simulink model "pendulo_invertido_bloque"  (R2025a)
settings: Solver=VariableStepAuto  StartTime=0.0  StopTime=10.0  RelTol=1e-3
PreLoadFcn:
  | % Parámetros físicos
  | Ip   = 0.0079;     % kg*m^2
  | Mc   = 0.7031;     % kg
  | lp   = 0.3302;     % m
  | lp2  = lp^2;       % m^2
  | lp3  = lp^3;       % m^3
  | Mp   = 0.23;       % kg
  | Mp2  = Mp^2;       % kg^2
  | Fc   = 0;          % N
  | Beq  = 4.3;        % Ns/m
  | g    = 9.81;       % m/s^2
  | Bp   = 0.0024;     % Nms/rad
  | 
  | % Condiciones iniciales de los estados
  | x       = 0;          % m
  | xdot      = 0;          % m/s
  | alpha   = 1*pi/180;   % rad
  | adot     = 0;          % rad/s
settings Model: Creator=Chris  LastModifiedBy=Chris

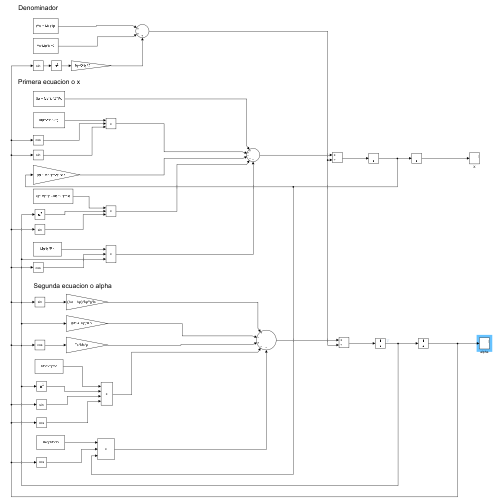
[thumbnail: Simulink's stored preview of the top-level diagram]
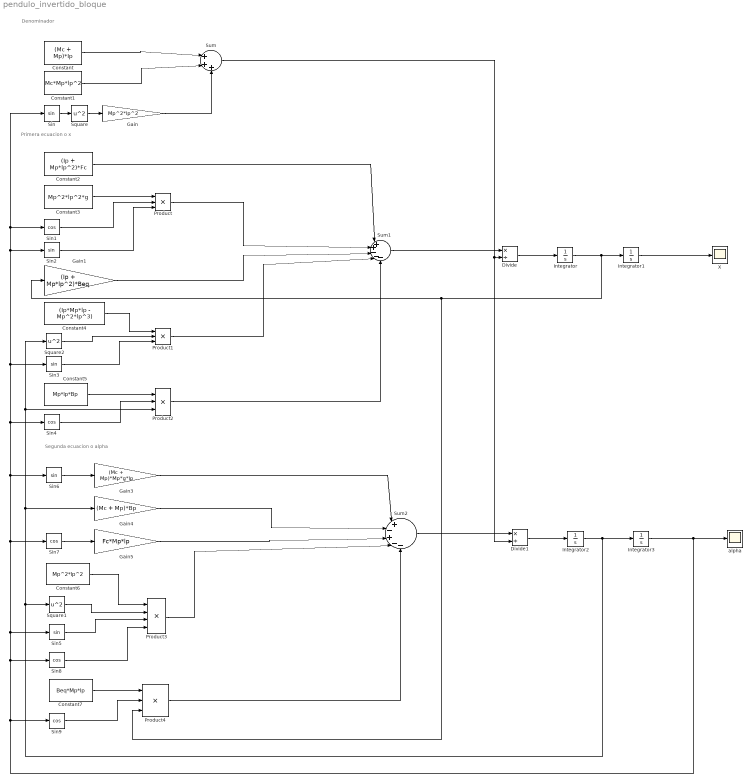
== system pendulo_invertido_bloque ==
  note: Segunda ecuacion o alpha
  note: Denominador
  note: Primera ecuacion o x
  Constant : Constant  Value=(Mc + Mp)*Ip
  Constant1 : Constant  Value=Mc*Mp*lp^2
  Constant2 : Constant  Value=(Ip + Mp*lp^2)*Fc
  Constant3 : Constant  Value=Mp^2*lp^2*g
  Constant4 : Constant  Value=(Ip*Mp*lp - Mp^2*lp^3)
  Constant5 : Constant  Value=Mp*lp*Bp
  Constant6 : Constant  Value=Mp^2*lp^2
  Constant7 : Constant  Value=Beq*Mp*lp
  Divide : Product  Inputs=*/
  Divide1 : Product  Inputs=*/
  Gain : Gain  Gain=Mp^2*lp^2
  Gain1 : Gain  Gain=(Ip + Mp*lp^2)*Beq
  Gain3 : Gain  Gain=(Mc + Mp)*Mp*g*lp
  Gain4 : Gain  Gain=(Mc + Mp)*Bp
  Gain5 : Gain  Gain=Fc*Mp*lp
  Integrator : Integrator
  Integrator1 : Integrator
  Integrator2 : Integrator
  Integrator3 : Integrator  InitialCondition=(1*pi)/180
  Product{,1..2,4} (4 alike) : Product  Inputs=3
  Product3 : Product  Inputs=4
  Sin{,2..3,5..6} (5 alike) : Trigonometry
  Sin{1,4,7..9} (5 alike) : Trigonometry  Operator=cos
  Square : Math  Operator=square
  Square1 : Math  Operator=square
  Square2 : Math  Operator=square
  Sum : Sum  Inputs=|+++
  Sum1 : Sum  Inputs=|++---
  Sum2 : Sum  Inputs=|+-+--
  X : Scope
      settings: ActiveDisplayYMinimum=-0.0043680008391681624  ActiveDisplayYMaximum=0.21434857965637735
  alpha : Scope
      settings: MaximizeAxes=On  ActiveDisplayYMinimum=-18.099425830783975  ActiveDisplayYMaximum=112.07325868766492
  wires:
  Constant/1 -> Sum/1
  Constant1/1 -> Sum/2
  Sin/1 -> Square/1
  Square/1 -> Gain/1
  Gain/1 -> Sum/3
  Constant2/1 -> Sum1/1
  Sin1/1 -> Product/2
  Constant3/1 -> Product/1
  Sin2/1 -> Product/3
  Product/1 -> Sum1/2
  Gain1/1 -> Sum1/3
  Constant4/1 -> Product1/1
  Square2/1 -> Product1/2
  Sin3/1 -> Product1/3
  Product1/1 -> Sum1/4
  Constant5/1 -> Product2/1
  Sin4/1 -> Product2/2
  Product2/1 -> Sum1/5
  Sin6/1 -> Gain3/1
  Sin7/1 -> Gain5/1
  Constant6/1 -> Product3/1
  Square1/1 -> Product3/2
  Sin5/1 -> Product3/3
  Sin8/1 -> Product3/4
  Constant7/1 -> Product4/1
  Sin9/1 -> Product4/2
  Gain3/1 -> Sum2/1
  Gain4/1 -> Sum2/2
  Gain5/1 -> Sum2/3
  Product3/1 -> Sum2/4
  Product4/1 -> Sum2/5
  Sum/1 -> Divide1/2, Divide/2
  Sum1/1 -> Divide/1
  Sum2/1 -> Divide1/1
  Divide/1 -> Integrator/1
  Integrator/1 -> Product4/3, Gain1/1, Integrator1/1
  Integrator1/1 -> X/1
  Divide1/1 -> Integrator2/1
  Integrator3/1 -> alpha/1, Sin9/1, Sin8/1, Sin5/1, Sin7/1, Sin6/1, Sin4/1, Sin3/1, Sin1/1, Sin/1, Sin2/1
  Integrator2/1 -> Integrator3/1, Square1/1, Gain4/1, Product2/3, Square2/1
